simulink model "flexibleDrive_NotchLeadLag"  (R2025b)
settings: Solver=ode4  StartTime=0.0  StopTime=4  FixedStep=Ts  RelTol=1e-3  EnableMultiTasking=on
values from neighbouring files (symbols this model uses):
  b1 = 0.003    [2_3_simulation.mat]
  b2 = 0.0003    [2_3_simulation.mat]
  C = 0    [2_3_simulation.mat]
  d1 = 0.4    [2_3_simulation.mat]
  d2 = 0.04    [2_3_simulation.mat]
  k = 0.07    [2_3_simulation.mat]
  m1 = 0.000551948051948    [2_3_simulation.mat]
  m2 = 0.000298051948052    [2_3_simulation.mat]
libraries: simulink x3
settings Model: Creator=user  LastModifiedBy=owenm
settings SolverCC: AlgebraicLoopSolver=TrustRegion
settings DataIOCC: ReturnWorkspaceOutputs=off
settings OptimizationCC: LifeSpan=inf
settings DebuggingCC: UnconnectedInputMsg=warning  UnconnectedOutputMsg=warning  UnconnectedLineMsg=warning  SFUnexpectedBacktrackingDiag=warning  SFNoUnconditionalDefaultTransitionDiag=warning  ArithmeticOperatorsInVariantConditions=warning
settings ModelReferenceCC: EnableRefExpFcnMdlSchedulingChecks=on
settings SFSimCC: SimUseLocalCustomCode=off  CustomCodeUndefinedFunction=UseInterfaceOnly
settings RTWCC: RTWUseLocalCustomCode=off  GPUComputeCapability=3.5  DLArmComputeVersion=19.05
settings CodeAppCC: StateflowObjectComments=on
settings GRTTargetCC: TargetLangStandard=C89/C90 (ANSI)
settings ConfigComp: CovMetricSettings=dw  CovSaveCumulativeToWorkspaceVar=on  CovSaveSingleToWorkspaceVar=on  CovExternalEMLEnable=off

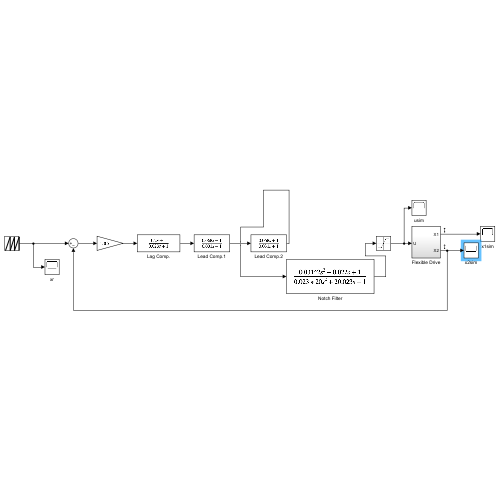
[thumbnail: Simulink's stored preview of the top-level diagram]
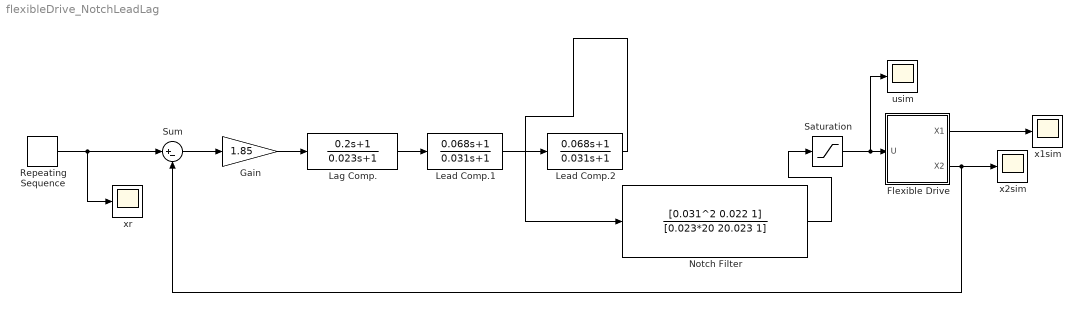
== system flexibleDrive_NotchLeadLag ==
  Flexible Drive : Subsystem
  Gain : Gain  Gain=1.85
  Lag Comp. : TransferFcn  Numerator=[0.2 1]  Denominator=[0.023 1]
  Lead Comp.1 : TransferFcn  Numerator=[ 0.068 1]  Denominator=[0.031 1]
  Lead Comp.2 : TransferFcn  Numerator=[ 0.068 1]  Denominator=[0.031 1]
  Notch Filter : TransferFcn  Numerator=[0.031^2 0.022 1]  Denominator=[0.023*20 20.023 1]
  Repeating Sequence : simulink/Sources/Repeating Sequence  rep_seq_t=time  rep_seq_y=s
  Saturation : Saturate  UpperLimit=8  LowerLimit=-8
  Sum : Sum  Inputs=|+-
  usim : Scope
      settings: ActiveDisplayYMinimum=-1.76239  ActiveDisplayYMaximum=1.76564  DataLoggingVariableName=usim
  x1sim : Scope
      settings: ActiveDisplayYMinimum=-57.411733886597688  ActiveDisplayYMaximum=102.34969324407008  DataLoggingVariableName=x1sim
  x2sim : Scope
      settings: ActiveDisplayYMinimum=-66.227174718096833  ActiveDisplayYMaximum=110.1500805667329  DataLoggingVariableName=x2sim
  xr : Scope
      settings: ActiveDisplayYMinimum=-6.25  ActiveDisplayYMaximum=56.25  DataLoggingVariableName=xr
  wires:
  Flexible Drive/1(X1) -> x1sim/1
  Flexible Drive/2(X2) -> x2sim/1, Sum/2
  Repeating Sequence/1 -> xr/1, Sum/1
  Notch Filter/1 -> Saturation/1
  Saturation/1 -> usim/1, Flexible Drive/1(U)
  Lead Comp.1/1 -> Lead Comp.2/1
  Lag Comp./1 -> Lead Comp.1/1
  Gain/1 -> Lag Comp./1
  Lead Comp.2/1 -> Notch Filter/1
  Sum/1 -> Gain/1

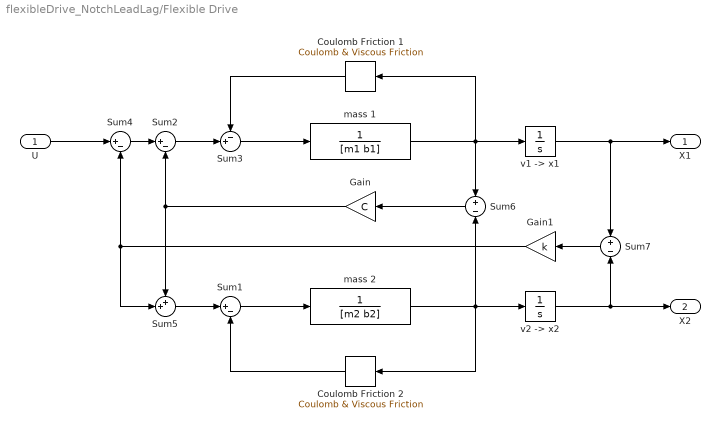
== system flexibleDrive_NotchLeadLag/Flexible Drive ==
  U : Inport
  Coulomb Friction 1 : simulink/Discontinuities/Coulomb & Viscous Friction  offset=[d1]  gain=0
  Coulomb Friction 2 : simulink/Discontinuities/Coulomb & Viscous Friction  offset=[d2]  gain=0
  Gain : Gain  Gain=C  SaturateOnIntegerOverflow=on  OutDataTypeStr=Inherit: Same as input  ParamDataTypeStr=Inherit: Same as input
  Gain1 : Gain  Gain=k  SaturateOnIntegerOverflow=on  OutDataTypeStr=Inherit: Same as input  ParamDataTypeStr=Inherit: Same as input
  Sum1 : Sum  Inputs=|+-  SaturateOnIntegerOverflow=on
  Sum2 : Sum  Inputs=|+-  SaturateOnIntegerOverflow=on
  Sum3 : Sum  Inputs=-+|  SaturateOnIntegerOverflow=on
  Sum4 : Sum  Inputs=|+-  SaturateOnIntegerOverflow=on
  Sum5 : Sum  Inputs=++|  SaturateOnIntegerOverflow=on
  Sum6 : Sum  Inputs=+|-  SaturateOnIntegerOverflow=on
  Sum7 : Sum  Inputs=+|-  SaturateOnIntegerOverflow=on
  mass 1 : TransferFcn  Denominator=[m1 b1]
  mass 2 : TransferFcn  Denominator=[m2 b2]
  "v1 -> x1" : Integrator
  "v2 -> x2" : Integrator
  X1 : Outport  VectorParamsAs1DForOutWhenUnconnected=off
  X2 : Outport  Port=2  VectorParamsAs1DForOutWhenUnconnected=off
  wires:
  Sum3/1 -> mass 1/1
  Sum1/1 -> mass 2/1
  Sum2/1 -> Sum3/2
  Sum6/1 -> Gain/1
  Gain/1 -> Sum2/2, Sum5/1
  "v1 -> x1"/1 -> Sum7/1, X1/1
  "v2 -> x2"/1 -> X2/1, Sum7/2
  Sum7/1 -> Gain1/1
  Gain1/1 -> Sum4/2, Sum5/2
  Sum4/1 -> Sum2/1
  U/1 -> Sum4/1
  mass 2/1 -> "v2 -> x2"/1, Coulomb Friction 2/1, Sum6/2
  Sum5/1 -> Sum1/1
  Coulomb Friction 1/1 -> Sum3/1
  mass 1/1 -> "v1 -> x1"/1, Coulomb Friction 1/1, Sum6/1
  Coulomb Friction 2/1 -> Sum1/2
